simulink model "control1_v3"  (R2015a)
settings: Solver=ode45  StartTime=0.0  StopTime=10.0  RelTol=1e-3
values from neighbouring files (symbols this model uses):
  g = param.g    [eq_quad.m]    (also in eq_quad_lin.m)
  m = param.m    [eq_quad.m]    (also in eq_quad_lin.m)
settings Model: Creator=jesus  LastModifiedBy=jesus

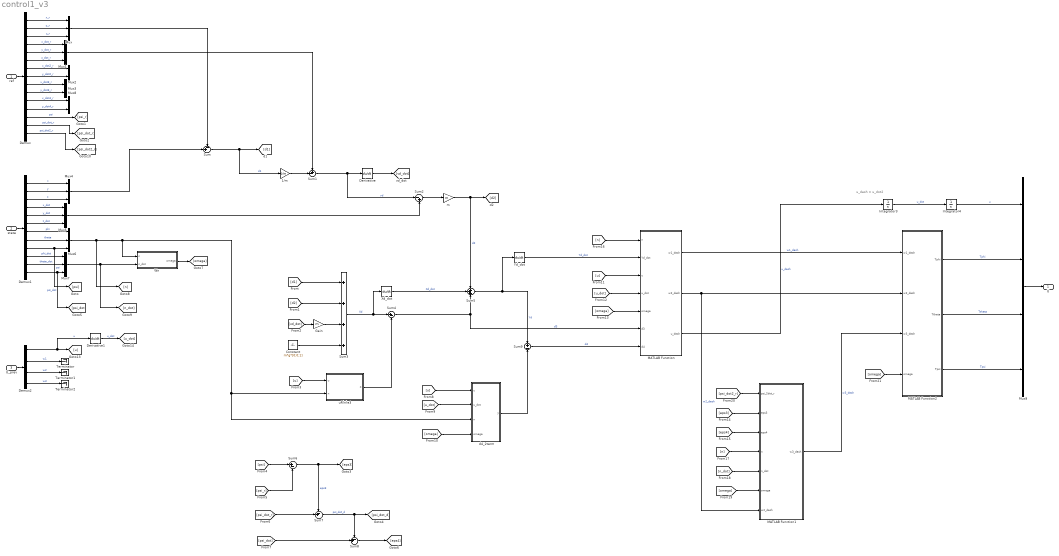
== system control1_v3 ==
  note: u_dash = u_dot2
  ref : Inport
  state : Inport  Port=2
  U_prev : Inport  Port=3
  1/m : Gain  Gain=1/m
  Constant : Constant  Value=m*g*[0;0;1]
  Demux : Demux  Outputs=15
  Demux1 : Demux  Outputs=12
  Demux2 : Demux
  Derivative : Derivative
  Derivative1 : Derivative
  Gain : Gain  Gain=m
  Integrator3 : Integrator
  Integrator4 : Integrator
  MATLAB Function : MATLAB Function  TreatAsAtomicUnit=on
  MATLAB Function1 : MATLAB Function  TreatAsAtomicUnit=on
  MATLAB Function2 : MATLAB Function  TreatAsAtomicUnit=on
  Mux{,1,4..7} (6 alike) : Mux  Inputs=3
  Mux2 : Mux  Inputs=2
  Mux3 : Mux  Inputs=2
  Mux8 : Mux  Inputs=2
  Mux9 : Mux
  Sum : Sum  Inputs=-+|
  Sum1 : Sum  Inputs=+-|
  Sum2 : Sum  Inputs=|-+
  Sum3 : Sum  Inputs=++++
  Sum4 : Sum  Inputs=|+-
  Sum5 : Sum  Inputs=+++
  Sum6 : Sum  Inputs=|+-
  Sum7 : Sum  Inputs=-+|
  Sum8 : Sum  Inputs=-+|
  Sum9 : Sum  Inputs=+|-
  Terminator : Terminator
  Terminator1 : Terminator
  Terminator2 : Terminator
  Wn : MATLAB Function  TreatAsAtomicUnit=on
  Xd_dot : Derivative
  Yd_dot : Derivative
  d4_2term : MATLAB Function  TreatAsAtomicUnit=on
  m : Gain  Gain=m
  uR(n)e3 : MATLAB Function  TreatAsAtomicUnit=on
  U : Outport
  wires:
  ref/1 -> Demux/1
  Demux/9 -> Mux3/1  "x_dot3_r"
  Demux/8 -> Mux2/2  "y_dot2_r"
  Demux/7 -> Mux2/1  "x_dot2_r"
  Demux/6 -> Mux1/3  "z_dot_r"
  Demux/5 -> Mux1/2  "y_dot_r"
  Demux/3 -> Mux/3  "z_r"
  Demux/2 -> Mux/2  "y_r"
  Demux/1 -> Mux/1  "x_r"
  Demux/12 -> Mux8/2  "y_dot4_r"
  Demux/4 -> Mux1/1  "x_dot_r"
  Demux1/1 -> Mux4/1  "x"
  Demux1/2 -> Mux4/2  "y"
  Demux1/3 -> Mux4/3  "z"
  Demux1/4 -> Mux5/1  "x_dot"
  state/1 -> Demux1/1
  Demux1/5 -> Mux5/2  "y_dot"
  Demux1/6 -> Mux5/3  "z_dot"
  Demux1/7 -> Mux6/1  "phi"
  Demux1/9 -> [psi], Mux6/3  "psi"
  Demux1/8 -> Mux6/2  "theta"
  Demux1/10 -> Mux7/1  "phi_dot"
  Demux1/11 -> Mux7/2  "theta_dot"
  Demux1/12 -> [psi_dot], Mux7/3  "psi_dot"
  Sum/1 -> 1/m/1, [d1]  "d1"
  Sum2/1 -> m/1
  Mux4/1 -> Sum/2
  Mux/1 -> Sum/1
  Mux1/1 -> Sum1/1
  1/m/1 -> Sum1/2
  Sum1/1 -> Sum2/1, Derivative/1  "vd"
  Mux5/1 -> Sum2/2
  m/1 -> [d2], Sum5/1  "d2"
  Derivative/1 -> [vd_dot]
  [vd_dot] -> Gain/1
  [d1] -> Sum3/1
  [d2] -> Sum3/2
  Gain/1 -> Sum3/3
  Constant/1 -> Sum3/4
  Sum3/1 -> Xd_dot/1, Sum4/1  "Xd"
  [u] -> uR(n)e3/1(u)
  uR(n)e3/1(X) -> Sum4/2
  Sum4/1 -> Sum5/3, MATLAB Function/6(d3)  "d3"
  Xd_dot/1 -> Sum5/2  "Xd_dot"
  Sum5/1 -> Sum9/1, Yd_dot/1  "Yd"
  [psi] -> Sum6/1
  [psi_r] -> Sum6/2
  Sum6/1 -> [eps3], Sum7/1  "eps3"
  [psi_dot_r] -> Sum7/2
  Sum7/1 -> [psi_dot_d], Sum8/1  "psi_dot_d"
  [psi_dot] -> Sum8/2
  Sum8/1 -> [eps4]
  Mux7/1 -> Wn/2(n_dot), [n_dot]
  Wn/1(omega) -> [omega]
  [u_dot] -> d4_2term/2(u_dot)
  [u] -> d4_2term/1(u)
  [omega] -> d4_2term/4(omega)
  Mux6/1 -> Wn/1(n), d4_2term/3(n), uR(n)e3/2(n), [n]
  d4_2term/1(y) -> Sum9/2
  Sum9/1 -> MATLAB Function/7(d4)  "d4"
  Yd_dot/1 -> MATLAB Function/2(Yd_dot)  "Yd_dot"
  [u_dot] -> MATLAB Function/4(u_dot)
  [u] -> MATLAB Function/3(u)
  [omega] -> MATLAB Function/5(omega)
  [eps3] -> MATLAB Function1/2(eps3)
  [eps4] -> MATLAB Function1/3(eps4)
  [n] -> MATLAB Function/1(n)
  [n] -> MATLAB Function1/4(n)
  [n_dot] -> MATLAB Function1/5(n_dot)
  [omega] -> MATLAB Function1/6(omega)
  MATLAB Function/2(w2_dash) -> MATLAB Function2/2(w2_dash), MATLAB Function1/7(w2_dash)  "w2_dash"
  Demux/10 -> Mux3/2  "y_dot3_r"
  Demux/11 -> Mux8/1  "x_dot4_r"
  Demux/13 -> [psi_r]  "psi"
  Demux/14 -> [psi_dot_r]  "psi_dot_r"
  Demux/15 -> [psi_dot2_r]  "psi_dot2_r"
  [psi_dot2_r] -> MATLAB Function1/1(psi_2dot_r)
  MATLAB Function/3(u_dash) -> Integrator3/1  "u_dash"
  Integrator3/1 -> Integrator4/1  "u_dot"
  Integrator4/1 -> Mux9/1  "u"
  U_prev/1 -> Demux2/1
  Demux2/2 -> Terminator/1  "w1"
  Demux2/3 -> Terminator1/1  "w2"
  Demux2/4 -> Terminator2/1  "w3"
  Mux9/1 -> U/1
  Demux2/1 -> Derivative1/1, [u]  "u"
  Derivative1/1 -> [u_dot]  "u_dot"
  MATLAB Function/1(w1_dash) -> MATLAB Function2/1(w1_dash)  "w1_dash"
  MATLAB Function1/1(w3_dash) -> MATLAB Function2/3(w3_dash)  "w3_dash"
  MATLAB Function2/1(Tphi) -> Mux9/2  "Tphi"
  MATLAB Function2/3(Tpsi) -> Mux9/4  "Tpsi"
  MATLAB Function2/2(Ttheta) -> Mux9/3  "Ttheta"
  [omega] -> MATLAB Function2/4(omega)

== matlab function control1_v3/Wn ==
  data: n input; omega output; n_dot input
function omega = Wn(n, n_dot)
% computes the angular velocities reative to the fixed frame

%inputs
phi = n(1);         theta = n(2);           psi = n(3);

% matrix Wn
    Wn = [ -sin(theta)           0         1
           cos(theta)*sin(psi)   cos(psi)  0
           cos(theta)*cos(psi)  -sin(psi)  0 ];
       
omega = Wn * n_dot;

== matlab function control1_v3/uR(n)e3 ==
  data: u input; X output; n input
function X = uRne3(u, n)
% Computes the lift force oriented along the axis Ea3 in the body fixed
%  frame {B}, principal force responsible to sustaining the quadcopter
%  flight.
%   X == Ea3 == u*R(n)*e3.

%Rotational matrix
    % angular/orientation states
    phi = n(1);  theta = n(2);   psi = n(3);
    % a = R(n)*e3
    a = [cos(phi)*sin(theta)*cos(psi)+sin(phi)*sin(psi)
         cos(phi)*sin(theta)*sin(psi)-sin(phi)*cos(psi)
         cos(phi)*cos(theta) ];

X = u * a;


% function R_n = R (n)
% % Computes the rotational matrix
% 
% % angular/orientation states
% phi = n(1);  theta = n(2);   psi = n(3);
% 
% R_n = [ cos(theta)*cos(psi)  sin(phi)*sin(theta)*cos(psi)-cos(phi)*sin(theta)  cos(phi)*sin(theta)*cos(psi)+sin(phi)*sin(psi)
%         cos(theta)*sin(phi)  sin(phi)*sin(theta)*sin(psi)+cos(phi)*cos(theta)  cos(phi)*sin(theta)*sin(psi)-sin(phi)*cos(psi) 
%         -sin(theta)          sin(phi)*cos(theta)                               cos(phi)*cos(theta)                           ];

== matlab function control1_v3/d4_2term ==
  data: u input; y output; u_dot input; n input; omega input
function y = d4_2term(u, u_dot, n, omega)
% Compute secind term for d4

% angular/orientation states
    phi = n(1);  theta = n(2);   psi = n(3);

    R_n = [ cos(theta)*cos(psi)  sin(phi)*sin(theta)*cos(psi)-cos(phi)*sin(psi)  cos(phi)*sin(theta)*cos(psi)+sin(phi)*sin(psi)
            cos(theta)*sin(psi)  sin(phi)*sin(theta)*sin(psi)+cos(phi)*cos(psi)  cos(phi)*sin(theta)*sin(psi)-sin(phi)*cos(psi) 
            -sin(theta)          sin(phi)*cos(theta)                               cos(phi)*cos(theta)                           ];

% skew simmetrix matrix of omega
    sk = [  0        -omega(3)  omega(2)
            omega(3)  0        -omega(1)
           -omega(2)  omega(1)  0       ];
e3 = [0;0;1];

y = u_dot*R_n*e3 + u*R_n*sk*e3;

== matlab function control1_v3/MATLAB Function ==
  data: n input; Yd_dot input; u input; w1_dash output; u_dot input; omega input; d3 input; d4 input; w2_dash output; u_dash output
function [w1_dash, w2_dash, u_dash] = fcn(n, Yd_dot, u, u_dot, omega, d3, d4)
% Computes equation (30) to obtain w1_dash, w2_dash, u_dash

% Right hand side of eq(30)
    % matrix R(n)
    phi = n(1); theta = n(2);   psi = n(3);
    
    R_n = [ cos(theta)*cos(psi)  sin(phi)*sin(theta)*cos(psi)-cos(phi)*sin(psi)  cos(phi)*sin(theta)*cos(psi)+sin(phi)*sin(psi)
            cos(theta)*sin(psi)  sin(phi)*sin(theta)*sin(psi)+cos(phi)*cos(psi)  cos(phi)*sin(theta)*sin(psi)-sin(phi)*cos(psi) 
            -sin(theta)          sin(phi)*cos(theta)                             cos(phi)*cos(theta)                           ];
    % skew simmetrix matrix of omega
    sk = [  0        -omega(3)  omega(2)
            omega(3)  0        -omega(1)
           -omega(2)  omega(1)  0       ];
    
    e3 = [0;0;1];
       
A = R_n' * ( Yd_dot - 2*u_dot*R_n*sk*e3 + d3 + d4 );
    
% Left hand side of eq(30) - asign values

    w1_dash = -A(1)/u;
    w2_dash =  A(2)/u;
    u_dash  =  A(3);

== matlab function control1_v3/MATLAB Function1 ==
  data: psi_2dot_r input; w3_dash output; eps3 input; eps4 input; n input; n_dot input; omega input; w2_dash input
function w3_dash = fcn(psi_2dot_r, eps3, eps4, n, n_dot, omega,w2_dash)
% Compute of equation (31) to obtain w3_dash

    e1 = [1;0;0];
    
    % orientation/angular states
    phi = n(1);          theta = n(2);          psi = n(3);
    phi_dot = n_dot(1);  theta_dot = n_dot(2);  psi_dot = n_dot(3);  
    % Wn_inv
    Wn_inv = [ 0           sin(phi)             cos(phi)
               0           cos(theta)*cos(phi) -cos(theta)*sin(phi)
               cos(theta)  sin(theta)*sin(phi)  sin(theta)*cos(phi) ];
    % Wn_dot
    Wn_dot = [ -cos(theta)*theta_dot                                        0                 0
               -sin(theta)*theta_dot*sin(phi)+cos(theta)*cos(phi)*phi_dot  -sin(phi)*phi_dot  0
               -sin(theta)*theta_dot*cos(phi)-cos(theta)*sin(phi)*phi_dot  -cos(phi)*phi-dot  0 ];
           
w3_dash = ( cos(theta)/cos(psi) ) * ( psi_2dot_r ...
                                    - eps4 ...
                                    - eps3 ...
                                    + e1' * Wn_inv * Wn_dot * Wn_inv * omega ...
                                    - ( sin(phi)/cos(theta) )*w2_dash );

== matlab function control1_v3/MATLAB Function2 ==
  data: w1_dash input; Tphi output; w2_dash input; w3_dash input; Ttheta output; Tpsi output; omega input
function [Tphi, Ttheta, Tpsi] = fcn(w1_dash, w2_dash, w3_dash, omega)
% Computes equation (26) to obtain the Torques in Euler's angles

% parameters
    global param
    Ix = param.Ix;  Iy = param.Iy;  Iz = param.Iz;
    QM = param.QM;  QT = param.QT;
    
    % P inertial matrix
    P = diag([Ix Iy Iz]);
    
w_dash = [ w1_dash; w2_dash; w3_dash ];


    % inv( eye(n) ) == eye(n)
    I = eye(3);
    
    e2 = [0;1;0];
    e3 = [0;0;1];
    
A = w_dash + cross(I*omega, I*omega) - QM*I*e3 + QT*I*e2;

w = inv(A)*w_dash;

% Torques in Euler's angles
Tphi = w(1);  Ttheta = w(2);  Tpsi = w(3);
